simulink model "pacemaker_with_serial_communication"  (R2020b)
settings: Solver=FixedStepAuto  StartTime=0.0  StopTime=10.0  FixedStep=1e-3  RelTol=1e-3  EnableMultiTasking=on
undefined symbols (not defined in the file): A0, A1, D0, D1, D10, D11, D12, D13, D2, D3, D4, D5, D6, D7, D8, D9, PTA0, PTA1, PTA2, PTB2, PTB23, PTB3, PTB9, PTC16, PTC17, PTC2, PTC3, PTC4, PTD0, PTD1, PTD2, PTD3
libraries: frdmk64flib x21, etargetslib x17
settings Model: ExtModeTrigDuration=5  Creator=Anna  LastModifiedBy=Nafi
settings OptimizationCC: EnhancedBackFolding=on  PassReuseOutputArgsAs=Individual arguments  ZeroExternalMemoryAtStartup=off  ZeroInternalMemoryAtStartup=off  MaxStackSize=64  OptimizeBlockOrder=speed  DifferentSizesBufferReuse=on  OptimizationCustomize=off  EfficientTunableParamExpr=on
settings DebuggingCC: ParameterTunabilityLossMsg=error
settings HardwareCC: ProdBitPerPointer=32  ProdBitPerSizeT=32  ProdBitPerPtrDiffT=32  ProdLargestAtomicInteger=Long  ProdLargestAtomicFloat=Double  ProdWordSize=32  ProdHWDeviceType=ARM Compatible->ARM Cortex
settings SFSimCC: MATLABDynamicMemAlloc=off
settings RTWCC: Description=Embedded Coder  SystemTargetFile=ert.tlc  HardwareBoard=NXP FRDM-K64F  TLCOptions="-aInlineSetEventsForThisBaseRateFcn=TLC_FALSE -aSuppressMultiTaskScheduler=TLC_FALSE  -aRateBasedStepFcn=0"  TemplateMakefile=ert_default_tmf  Toolchain=GNU Tools for ARM Embedded Processors
settings CodeAppCC: ForceParamTrailComments=on  IgnoreCustomStorageClasses=off  OperatorAnnotations=on  SimulinkDataObjDesc=on  SFDataObjDesc=on  InsertBlockDesc=on
settings ERTTargetCC: ExtModeTransport=4  ExtModeMexFile=sendToCommService

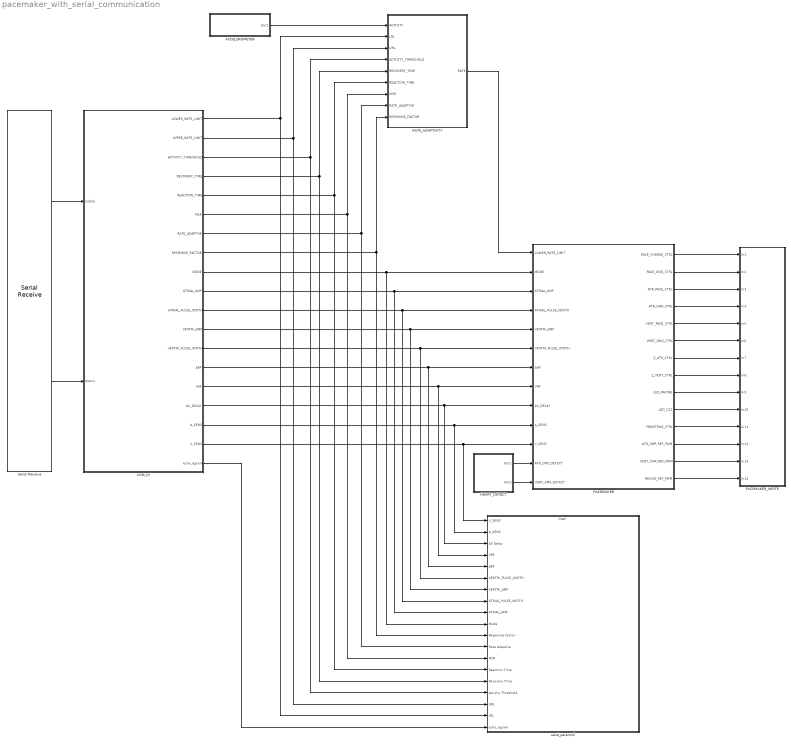
== system pacemaker_with_serial_communication ==
  ACCELEROMETER : Subsystem
  COM_IN : Stateflow chart  TreatAsAtomicUnit=on
      settings: PortSchema="{\"entries\":[{\"content\":{\"sides\":[{\"content\":{\"connectorIds\":[\"In1\",\"In2\"]},\"type\":\"ConnectorPlacement.EquallySpacedRectSide\",\"uuid\":\"cd1265d4-eeab-406f-839b-31637b64935e\"},{\"content\":{\"connectorIds\":[\"Out1\",\"Out2\",\"Out3\",\"Out4\",\"Out5\",\"Out6\",\"Out7\",\"Out8\",\"Out11\",\"Out15\",\"Out18\",\"Out16\",\"Out17\",\"Out10\",\"Out9\",\"Out13\",\"Out12\",\"Out14\",\"Out19\"],\"side\":\"RIGHT\"},\"type\":\"ConnectorPlacement.EquallySpacedRectSide\",\"uuid\":\"4c8a5d3b-ca50-43d3-bdc9-bcde3c420f64\"},{\"content\":{\"connectorIds\":[],\"side\":\"TOP\"},\"type\":\"ConnectorPlacement.EquallySpacedRectSide\",\"uuid\":\"7503811e-7a3c-4f49-863d-267d8f14587a\"},{\"content\":{\"connectorIds\":[],\"side\":\"HIDDEN\"},\"type\":\"ConnectorPlacement.EquallySpacedRectSide\",\"uuid\":\"b2e57f36-2a2e-483e-a972-25b3276b1e9d\"}]},\"type\":\"ConnectorPlacement.EquallySpacedConnector\",\"uuid\":\"ec734eff-85b8-4214-815d-279c5f21987a\"}],\"packageUris\":[\"http://schema.mathworks.com/mf0/Connector/R2020b\"],\"version\":\"1.0\"}"
  HEART_DETECT : Subsystem
  PACEMAKER : Stateflow chart  TreatAsAtomicUnit=on
      settings: PortSchema="{\"entries\":[{\"content\":{\"sides\":[{\"content\":{\"connectorIds\":[\"In2\",\"In1\",\"In3\",\"In4\",\"In5\",\"In6\",\"In7\",\"In8\",\"In9\",\"In10\",\"In11\",\"In12\",\"In13\"]},\"type\":\"ConnectorPlacement.EquallySpacedRectSide\",\"uuid\":\"703ea547-b5e3-494b-9c56-53f76044caab\"},{\"content\":{\"connectorIds\":[\"Out1\",\"Out2\",\"Out3\",\"Out4\",\"Out5\",\"Out6\",\"Out7\",\"Out8\",\"Out9\",\"Out10\",\"Out11\",\"Out12\",\"Out13\",\"Out14\"],\"side\":\"RIGHT\"},\"type\":\"ConnectorPlacement.EquallySpacedRectSide\",\"uuid\":\"cc2727a3-7e1d-4420-9643-b4757eb365ba\"},{\"content\":{\"connectorIds\":[],\"side\":\"TOP\"},\"type\":\"ConnectorPlacement.EquallySpacedRectSide\",\"uuid\":\"492b7801-5c9e-4474-b04e-880113f9bc08\"},{\"content\":{\"connectorIds\":[],\"side\":\"HIDDEN\"},\"type\":\"ConnectorPlacement.EquallySpacedRectSide\",\"uuid\":\"c524ea30-cb2c-406f-8230-58907bd7faf1\"}]},\"type\":\"ConnectorPlacement.EquallySpacedConnector\",\"uuid\":\"90428471-58b8-4273-9dd0-f9ed52ecca6a\"}],\"packageUris\":[\"http://schema.mathworks.com/mf0/Connector/R2020b\"],\"version\":\"1.0\"}"
  PACEMAKER_WRITE : Subsystem
  RATE_ADAPTIVITY : Stateflow chart  TreatAsAtomicUnit=on
      settings: PortSchema="{\"entries\":[{\"content\":{\"sides\":[{\"content\":{\"connectorIds\":[\"In1\",\"In2\",\"In3\",\"In4\",\"In6\",\"In5\",\"In7\",\"In8\",\"In9\"]},\"type\":\"ConnectorPlacement.EquallySpacedRectSide\",\"uuid\":\"d09d22a4-3bf2-447a-b888-9ed1bc13e508\"},{\"content\":{\"connectorIds\":[\"Out1\"],\"side\":\"RIGHT\"},\"type\":\"ConnectorPlacement.EquallySpacedRectSide\",\"uuid\":\"e5a6e6ed-c47a-4985-9dbc-dfef5f432796\"},{\"content\":{\"connectorIds\":[],\"side\":\"TOP\"},\"type\":\"ConnectorPlacement.EquallySpacedRectSide\",\"uuid\":\"14194fe3-110c-41d4-af12-2dfde4f1ce34\"},{\"content\":{\"connectorIds\":[],\"side\":\"HIDDEN\"},\"type\":\"ConnectorPlacement.EquallySpacedRectSide\",\"uuid\":\"89c167d3-ea6f-444e-9874-109804893e2e\"}]},\"type\":\"ConnectorPlacement.EquallySpacedConnector\",\"uuid\":\"492e352f-68f6-4e08-ae59-46af104c6e80\"}],\"packageUris\":[\"http://schema.mathworks.com/mf0/Connector/R2020b\"],\"version\":\"1.0\"}"
  Serial Receive : frdmk64flib/Serial Receive  SCIModule=0  Baudrate=uint32(9600)  Parity=None  StopBits=1  HardwareFlowControl=None  ByteOrder=LittleEndian  DataType=uint8  DataLength=52  BlockingMode=off  OutputStatus=on  SampleTime=0.015
  send_params() : Subsystem
  wires:
  COM_IN/17(VENTRI_PULSE_WIDTH) -> send_params()/6(VENTRI_PULSE_WIDTH), PACEMAKER/6(VENTRI_PULSE_WIDTH)
  COM_IN/10(ARP) -> send_params()/5(ARP), PACEMAKER/7(ARP)
  COM_IN/18(ATRIAL_PULSE_WIDTH) -> send_params()/8(ATRIAL_PULSE_WIDTH), PACEMAKER/4(ATRIAL_PULSE_WIDTH)
  COM_IN/12(A_SENS) -> send_params()/2(A_SENS), PACEMAKER/10(A_SENS)
  COM_IN/9(VRP) -> send_params()/4(VRP), PACEMAKER/8(VRP)
  COM_IN/1(LOWER_RATE_LIMIT) -> send_params()/18(LRL), RATE_ADAPTIVITY/2(LRL)
  COM_IN/13(AV_DELAY) -> send_params()/3(AV Delay), PACEMAKER/9(AV_DELAY)
  COM_IN/14(V_SENS) -> send_params()/1(V_SENS), PACEMAKER/11(V_SENS)
  COM_IN/11(MODE) -> send_params()/10(Mode), PACEMAKER/1(MODE)
  COM_IN/3(ACTIVITY_THRESHOLD) -> send_params()/16(Activity Threshold), RATE_ADAPTIVITY/4(ACTIVITY_THRESHOLD)
  COM_IN/6(MSR) -> send_params()/13(MSR), RATE_ADAPTIVITY/7(MSR)
  COM_IN/2(UPPER_RATE_LIMIT) -> send_params()/17(URL), RATE_ADAPTIVITY/3(URL)
  PACEMAKER/3(ATR_PACE_CTRL) -> PACEMAKER_WRITE/3(In3)
  COM_IN/7(RATE_ADAPTIVE) -> send_params()/12(Rate Adaptive), RATE_ADAPTIVITY/8(RATE_ADAPTIVE)
  RATE_ADAPTIVITY/1(RATE) -> PACEMAKER/2(LOWER_RATE_LIMIT)
  Serial Receive/2 -> COM_IN/2(status)
  PACEMAKER/9(LED_PACING) -> PACEMAKER_WRITE/9(In9)
  Serial Receive/1 -> COM_IN/1(rxdata)
  COM_IN/15(ATRIAL_AMP) -> send_params()/9(ATRIAL_AMP), PACEMAKER/3(ATRIAL_AMP)
  PACEMAKER/11(FRONTEND_CTRL) -> PACEMAKER_WRITE/11(In11)
  PACEMAKER/12(ATR_CMP_REF_PWM) -> PACEMAKER_WRITE/12(In12)
  PACEMAKER/1(PACE_CHARGE_CTRL) -> PACEMAKER_WRITE/1(In1)
  PACEMAKER/7(Z_ATR_CTRL) -> PACEMAKER_WRITE/7(In7)
  PACEMAKER/5(VENT_PACE_CTRL) -> PACEMAKER_WRITE/5(In5)
  PACEMAKER/10(LED_C22) -> PACEMAKER_WRITE/10(In10)
  PACEMAKER/2(PACE_GND_CTRL) -> PACEMAKER_WRITE/2(In2)
  PACEMAKER/14(PACING_REF_PWM) -> PACEMAKER_WRITE/14(In14)
  HEART_DETECT/2(Out2) -> PACEMAKER/13(VENT_CMP_DETECT)
  PACEMAKER/6(VENT_GND_CTRL) -> PACEMAKER_WRITE/6(In6)
  COM_IN/8(RESPONSE_FACTOR) -> send_params()/11(Response Factor), RATE_ADAPTIVITY/9(RESPONSE_FACTOR)
  PACEMAKER/4(ATR_GND_CTRL) -> PACEMAKER_WRITE/4(In4)
  COM_IN/5(REACTION_TIME) -> send_params()/14(Reaction Time), RATE_ADAPTIVITY/5(REACTION_TIME)
  COM_IN/16(VENTRI_AMP) -> send_params()/7(VENTRI_AMP), PACEMAKER/5(VENTRI_AMP)
  PACEMAKER/8(Z_VENT_CTRL) -> PACEMAKER_WRITE/8(In8)
  PACEMAKER/13(VENT_CMP_REF_PWM) -> PACEMAKER_WRITE/13(In13)
  COM_IN/4(RECOVERY_TIME) -> send_params()/15(Recovery Time), RATE_ADAPTIVITY/6(RECOVERY_TIME)
  HEART_DETECT/1(Out1) -> PACEMAKER/12(ATR_CMP_DETECT)
  COM_IN/19(echo_egram) -> send_params()/19(echo_egram)
  ACCELEROMETER/1(Out1) -> RATE_ADAPTIVITY/1(ACTIVITY)

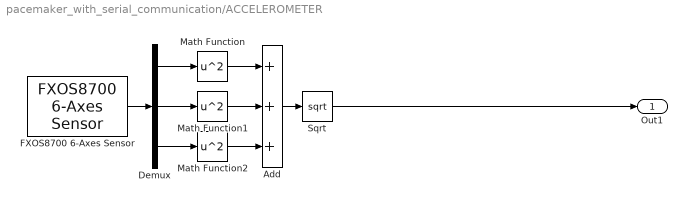
== system pacemaker_with_serial_communication/ACCELEROMETER ==
  Add : Sum  Inputs=+++
  Demux : Demux  Outputs=3
  FXOS8700 6-Axes Sensor : frdmk64flib/FXOS8700 6-Axes Sensor  Activesensor=Accelerometer only  ODR=800Hz  HybridODR=400Hz  Accelfullrange=-4g to +4g  SampleTime=-1
  Math Function : Math  Operator=square  SaturateOnIntegerOverflow=on
  Math Function1 : Math  Operator=square  SaturateOnIntegerOverflow=on
  Math Function2 : Math  Operator=square  SaturateOnIntegerOverflow=on
  Sqrt : Sqrt  SaturateOnIntegerOverflow=on
  Out1 : Outport
  wires:
  Add/1 -> Sqrt/1
  Demux/2 -> Math Function1/1
  Demux/3 -> Math Function2/1
  FXOS8700 6-Axes Sensor/1 -> Demux/1
  Demux/1 -> Math Function/1
  Math Function2/1 -> Add/3
  Sqrt/1 -> Out1/1
  Math Function/1 -> Add/1
  Math Function1/1 -> Add/2

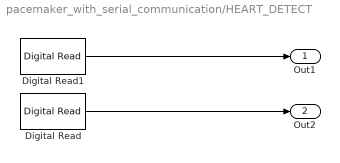
== system pacemaker_with_serial_communication/HEART_DETECT ==
  Digital Read : frdmk64flib/Digital Read  Whichpin=PTC17 (D1)  SampleTime=-1
  Digital Read1 : frdmk64flib/Digital Read  Whichpin=PTC16 (D0)  SampleTime=-1
  Out1 : Outport
  Out2 : Outport  Port=2
  wires:
  Digital Read/1 -> Out2/1
  Digital Read1/1 -> Out1/1

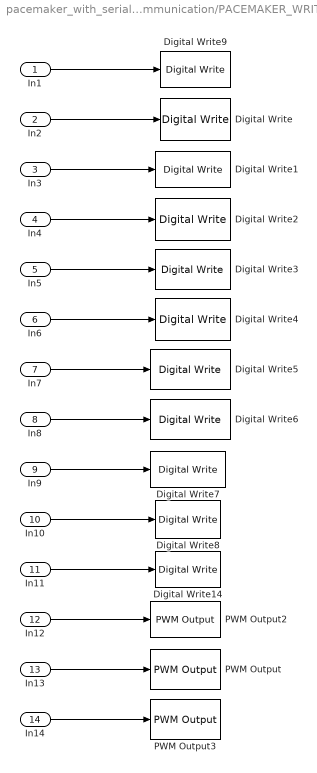
== system pacemaker_with_serial_communication/PACEMAKER_WRITE ==
  In1 : Inport
  In2 : Inport  Port=2
  In3 : Inport  Port=3
  In4 : Inport  Port=4
  In5 : Inport  Port=5
  In6 : Inport  Port=6
  In7 : Inport  Port=7
  In8 : Inport  Port=8
  In9 : Inport  Port=9
  In10 : Inport  Port=10
  In11 : Inport  Port=11
  In12 : Inport  Port=12
  In13 : Inport  Port=13
  In14 : Inport  Port=14
  Digital Write : frdmk64flib/Digital Write  Whichpin=PTD0 (D10)
  Digital Write1 : frdmk64flib/Digital Write  Whichpin=PTA0 (D8)
  Digital Write14 : frdmk64flib/Digital Write  Whichpin=PTD1 (D13)
  Digital Write2 : frdmk64flib/Digital Write  Whichpin=PTD2 (D11)
  Digital Write3 : frdmk64flib/Digital Write  Whichpin=PTC4 (D9)
  Digital Write4 : frdmk64flib/Digital Write  Whichpin=PTD3 (D12)
  Digital Write5 : frdmk64flib/Digital Write  Whichpin=PTB23 (D4)
  Digital Write6 : frdmk64flib/Digital Write  Whichpin=PTC3 (D7)
  Digital Write7 : frdmk64flib/Digital Write  Whichpin=RED_LED
  Digital Write8 : frdmk64flib/Digital Write  Whichpin=BLUE_LED
  Digital Write9 : frdmk64flib/Digital Write  Whichpin=PTB9 (D2)
  PWM Output : frdmk64flib/PWM Output  Whichpin=PTA1 (D3)  InitialFrequency=2000  InitialDutyCycle=100
  PWM Output2 : frdmk64flib/PWM Output  Whichpin=PTC2 (D6)  InitialFrequency=2000  InitialDutyCycle=100
  PWM Output3 : frdmk64flib/PWM Output  Whichpin=PTA2 (D5)  InitialFrequency=2000  InitialDutyCycle=100
  wires:
  In10/1 -> Digital Write8/1
  In2/1 -> Digital Write/1
  In12/1 -> PWM Output2/1
  In7/1 -> Digital Write5/1
  In4/1 -> Digital Write2/1
  In8/1 -> Digital Write6/1
  In11/1 -> Digital Write14/1
  In1/1 -> Digital Write9/1
  In6/1 -> Digital Write4/1
  In9/1 -> Digital Write7/1
  In14/1 -> PWM Output3/1
  In3/1 -> Digital Write1/1
  In13/1 -> PWM Output/1
  In5/1 -> Digital Write3/1

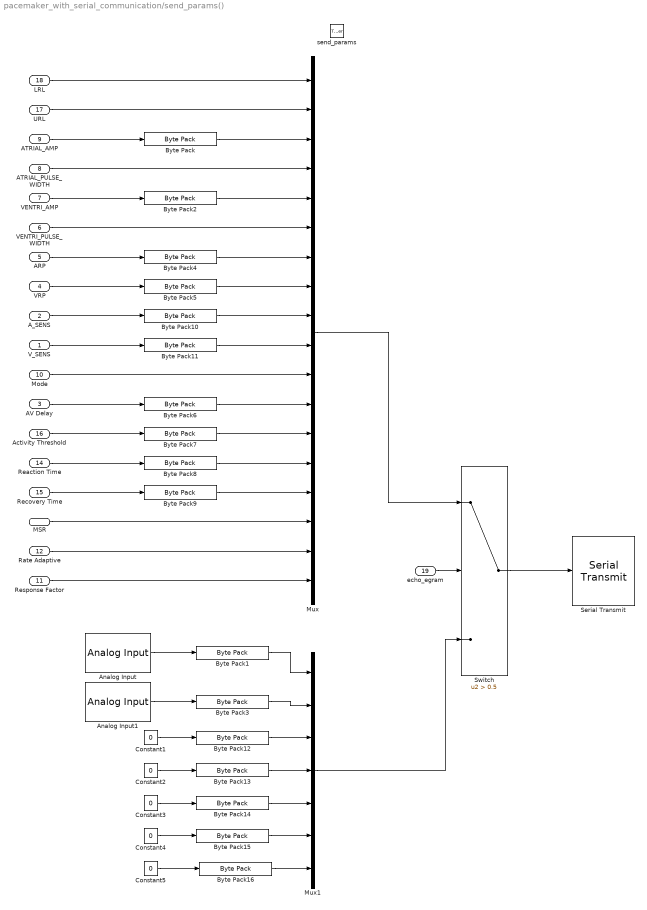
== system pacemaker_with_serial_communication/send_params() ==
  V_SENS : Inport
  A_SENS : Inport  Port=2
  AV Delay : Inport  Port=3
  VRP : Inport  Port=4
  ARP : Inport  Port=5
  VENTRI_PULSE_WIDTH : Inport  Port=6
  VENTRI_AMP : Inport  Port=7
  ATRIAL_PULSE_WIDTH : Inport  Port=8
  ATRIAL_AMP : Inport  Port=9
  Mode : Inport  Port=10
  Response Factor : Inport  Port=11
  Rate Adaptive : Inport  Port=12
  MSR : Inport  Port=13
  Reaction Time : Inport  Port=14
  Recovery Time : Inport  Port=15
  Activity Threshold : Inport  Port=16
  URL : Inport  Port=17
  LRL : Inport  Port=18
  echo_egram : Inport  Port=19
  send_params : TriggerPort  TriggerType=function-call  IsSimulinkFunction=on  FunctionName=send_params  VariantControl=Variant
  Analog Input : frdmk64flib/Analog Input  Whichpin=PTB2 (A0)  SampleTime=-1
  Analog Input1 : frdmk64flib/Analog Input  Whichpin=PTB3 (A1)  SampleTime=-1
  Byte Pack{,2,7,10..11} (5 alike) : etargetslib/Byte Pack  datatypes={'single'}  byteAlign=1
  Byte Pack{1,3,8..9,12..15} (8 alike) : etargetslib/Byte Pack  datatypes={'double'}  byteAlign=1
  Byte Pack{4..6,16} (4 alike) : etargetslib/Byte Pack  datatypes={'uint16'}  byteAlign=1
  Constant{1..4} (4 alike) : Constant  Value=0  OutDataTypeStr=double
  Constant5 : Constant  Value=0  OutDataTypeStr=uint16
  Mux : Mux  Inputs=18
  Mux1 : Mux  Inputs=7
  Serial Transmit : frdmk64flib/Serial Transmit  SCIModule=0  Baudrate=uint32(9600)  Parity=None  StopBits=1  HardwareFlowControl=None  ByteOrder=LittleEndian  BlockingMode=on  OutputStatus=off
  Switch : Switch  Criteria=u2 > Threshold  Threshold=0.5
  wires:
  LRL/1 -> Mux/1
  URL/1 -> Mux/2
  ATRIAL_AMP/1 -> Byte Pack/1
  VENTRI_AMP/1 -> Byte Pack2/1
  ARP/1 -> Byte Pack4/1
  VRP/1 -> Byte Pack5/1
  A_SENS/1 -> Byte Pack10/1
  AV Delay/1 -> Byte Pack6/1
  Activity Threshold/1 -> Byte Pack7/1
  Reaction Time/1 -> Byte Pack8/1
  Recovery Time/1 -> Byte Pack9/1
  Byte Pack/1 -> Mux/3
  ATRIAL_PULSE_WIDTH/1 -> Mux/4
  Byte Pack2/1 -> Mux/5
  VENTRI_PULSE_WIDTH/1 -> Mux/6
  Byte Pack4/1 -> Mux/7
  Byte Pack5/1 -> Mux/8
  V_SENS/1 -> Byte Pack11/1
  Byte Pack10/1 -> Mux/9
  Analog Input/1 -> Byte Pack1/1
  Analog Input1/1 -> Byte Pack3/1
  Constant1/1 -> Byte Pack12/1
  Constant2/1 -> Byte Pack13/1
  Constant3/1 -> Byte Pack14/1
  Constant4/1 -> Byte Pack15/1
  Constant5/1 -> Byte Pack16/1
  Byte Pack15/1 -> Mux1/6
  Byte Pack14/1 -> Mux1/5
  Byte Pack13/1 -> Mux1/4
  Byte Pack12/1 -> Mux1/3
  Byte Pack1/1 -> Mux1/1
  Byte Pack3/1 -> Mux1/2
  echo_egram/1 -> Switch/2
  Mux1/1 -> Switch/3
  Mux/1 -> Switch/1
  Switch/1 -> Serial Transmit/1
  Byte Pack16/1 -> Mux1/7
  Byte Pack11/1 -> Mux/10
  Mode/1 -> Mux/11
  Byte Pack9/1 -> Mux/15
  Byte Pack6/1 -> Mux/12
  Byte Pack7/1 -> Mux/13
  Byte Pack8/1 -> Mux/14
  MSR/1 -> Mux/16
  Rate Adaptive/1 -> Mux/17
  Response Factor/1 -> Mux/18

== stateflow chart pacemaker_with_serial_communication/COM_IN ==
  settings: executeAtInitialization=1
  state SET_PARAMS
    entry:
    LOWER_RATE_LIMIT = rxdata(3)
    UPPER_RATE_LIMIT = rxdata(4)
    ATRIAL_AMP = typecast(rxdata(5:8), 'single')
    ATRIAL_PULSE_WIDTH = rxdata(9)
    VENTRI_AMP = typecast(rxdata(10:13), 'single')
    VENTRI_PULSE_WIDTH = rxdata(14)
    ARP = typecast(rxdata(15:16), 'uint16')
    VRP = typecast(rxdata(17:18), 'uint16')
    A_SENS = typecast(rxdata(19:22), 'single')
    V_SENS = typecast(rxdata(23:26), 'single')
    MODE = rxdata(27)
    AV_DELAY = typecast(rxdata(28:29),'uint16')
    ACTIVITY_THRESHOLD = typecast(rxdata(30:33), 'single')
    REACTION_TIME = typecast(rxdata(34:41), 'double')
    RECOVERY_TIME = typecast(rxdata(42:49), 'double')
    MSR = rxdata(50)
    RATE_ADAPTIVE = rxdata(51)
    RESPONSE_FACTOR= rxdata(52)
  state INIT
    entry:
    LOWER_RATE_LIMIT = 30
    UPPER_RATE_LIMIT = 120
    ATRIAL_AMP = 5
    ATRIAL_PULSE_WIDTH = 10
    VENTRI_AMP = 5
    VENTRI_PULSE_WIDTH = 10
    ARP = 100
    VRP = 100
    A_SENS= 3
    V_SENS = 3
    MODE = 4
    AV_DELAY = 50
    ACTIVITY_THRESHOLD = 1.1
    REACTION_TIME = 2000
    RECOVERY_TIME = 2000
    MSR = 120
    RATE_ADAPTIVE= 1
    RESPONSE_FACTOR = 16
  state SEND_EGRAM
    entry:
    echo_egram = 0
    send_params()
  state STANDBY
  state SEND_PARAMS
    entry:
    echo_egram = 1
    send_params();
  SET_PARAMS -> STANDBY
  (junction 10) -> SET_PARAMS [order 2] : [rxdata(2) == hex2dec('55')]
  (default) -> INIT
  INIT -> STANDBY
  STANDBY -> (junction 10) : [status == 0 && rxdata(1) == hex2dec('16')]
  (junction 10) -> SEND_EGRAM [order 1] : [rxdata(2) == hex2dec('47')]
  (junction 10) -> SEND_PARAMS [order 3] : [rxdata(2) == hex2dec('22')]
  SEND_EGRAM -> STANDBY
  SEND_PARAMS -> STANDBY
  data: LOWER_RATE_LIMIT output uint8; rxdata input uint8; status input uint8; UPPER_RATE_LIMIT output uint8; ACTIVITY_THRESHOLD output single; RECOVERY_TIME output double; REACTION_TIME output double; MSR output uint8; RATE_ADAPTIVE output uint8; RESPONSE_FACTOR output uint8; VRP output uint16; ARP output uint16; MODE output uint8; A_SENS output single; AV_DELAY output uint16; V_SENS output single; ATRIAL_AMP output single; VENTRI_AMP output single; VENTRI_PULSE_WIDTH output uint8; ATRIAL_PULSE_WIDTH output uint8; echo_egram output

== stateflow chart pacemaker_with_serial_communication/RATE_ADAPTIVITY ==
  state MIN_RATE
    AVG_ACTIVITY = (AVG_ACTIVITY + ACTIVITY)/2
    if RATE > LRL
    RATE = RATE - (MSR-LRL)/RECOVERY_TIME
    DELAY = RECOVERY_TIME
    else
    RATE = LRL
    DELAY = 0
    end
  state INITIAL
    RATE = LRL
    AVG_ACTIVITY = ACTIVITY
  state RATE_ADAPTIVE_DEFAULT
  state RATE_ADAPTIVE
    ADJUSTED_RATE = (0.57*RESPONSE_FACTOR^2-1.34*RESPONSE_FACTOR+22.71)*(AVG_ACTIVITY- double(ACTIVITY_THRESHOLD))+LRL
    if ADJUSTED_RATE > MSR
    ADJUSTED_RATE = MSR
    elseif ADJUSTED_RATE < LRL
    ADJUSTED_RATE = LRL
    end
  state OFFSET
    AVG_ACTIVITY = (AVG_ACTIVITY + ACTIVITY)/2
    if RATE > ADJUSTED_RATE
    RATE = RATE - (MSR-LRL)/RECOVERY_TIME
    DELAY = RECOVERY_TIME
    elseif RATE < ADJUSTED_RATE
    RATE = RATE + (MSR-LRL)/REACTION_TIME
    DELAY = REACTION_TIME
    end
  MIN_RATE -> RATE_ADAPTIVE [order 1] : [n>= DELAY && AVG_ACTIVITY>=ACTIVITY_THRESHOLD]
  MIN_RATE -> MIN_RATE [order 2] : after(1,msec){n=n+1}
  MIN_RATE -> INITIAL [order 3] : [RATE_ADAPTIVE == 0 && n>=DELAY]
  RATE_ADAPTIVE_DEFAULT -> MIN_RATE [order 2] : [AVG_ACTIVITY < double(ACTIVITY_THRESHOLD)]{n=0}
  (default) -> INITIAL
  INITIAL -> RATE_ADAPTIVE_DEFAULT : [RATE_ADAPTIVE == 1]{ADJUSTED_RATE = RATE}
  RATE_ADAPTIVE_DEFAULT -> RATE_ADAPTIVE [order 1] : [AVG_ACTIVITY>= ACTIVITY_THRESHOLD]
  OFFSET -> RATE_ADAPTIVE_DEFAULT [order 1] : [n>=DELAY]
  RATE_ADAPTIVE -> OFFSET : {n=0, AVG_ACTIVITY = ACTIVITY}
  OFFSET -> OFFSET [order 2] : after(1, msec){n=n+1}
  data: ACTIVITY input; LRL input uint8; RATE output; URL input uint8; ACTIVITY_THRESHOLD input single; REACTION_TIME input double; RECOVERY_TIME input double; MSR input uint8; BPM_PREV local; CURRENT_BPM local; PREV_ACCEL local; n local; AVG_ACCEL local; RATE_ADAPTIVE input uint8; RESPONSE_FACTOR input uint8; ADJUSTED_RATE local; AVG_ACTIVITY local; DELAY local

== stateflow chart pacemaker_with_serial_communication/PACEMAKER ==
  state MODE_VVI [commented out]
    entry:
    FRONTEND_CTRL = true
    state VVI_CHARGING_SENSING [commented out]
      entry:
      %Sensing Circuitry
      VENT_CMP_REF_PWM = DUTY_CYCLE
      ATR_CMP_REF_PWM = 0
      %Discharging C21
      PACE_GND_CTRL = true
      VENT_PACE_CTRL = false
      Z_ATR_CTRL = false
      Z_VENT_CTRL = false
      ATR_PACE_CTRL = false
      ATR_GND_CTRL = false
      VENT_GND_CTRL = true
      %Charging C22
      ATR_PACE_CTRL = false
      VENT_PACE_CTRL = false
      PACING_REF_PWM = 100*VENTRI_AMP/5
      PACE_CHARGE_CTRL = true
      LED_C22 = true
      exit:
      LED_C22 = false
    state PACE_READY [commented out]
      entry:
      %Discharging C21
      PACE_GND_CTRL = true
      VENT_PACE_CTRL = false
      Z_ATR_CTRL = false
      Z_VENT_CTRL = false
      ATR_PACE_CTRL = false
      ATR_GND_CTRL = false
      VENT_GND_CTRL = true
      %Charging C22
      ATR_PACE_CTRL = false
      VENT_PACE_CTRL = false
      PACING_REF_PWM = 100*VENTRI_AMP/5
      PACE_CHARGE_CTRL = true
      LED_C22 = true
      exit:
      LED_C22 = false
    state PACING_VENTRICLE_VVI [commented out]
      entry:
      PACE_CHARGE_CTRL = false
      PACE_GND_CTRL = true
      ATR_PACE_CTRL = false
      ATR_GND_CTRL = false
      Z_ATR_CTRL = false
      Z_VENT_CTRL = false
      VENT_GND_CTRL = false
      VENT_PACE_CTRL = true
      LED_PACING = true
      exit:
      LED_PACING = false
    VVI_CHARGING_SENSING -> PACING_VENTRICLE_VVI [commented out] : after(((60000/LOWER_RATE_LIMIT)-VENTRI_PULSE_WIDTH-VRP),msec) [VENT_CMP_DETECT== false]
    (default) -> VVI_CHARGING_SENSING [commented out]
    MODE_VVI.PACE_READY -> VVI_CHARGING_SENSING [commented out] : after(VRP, msec)
    PACING_VENTRICLE_VVI -> MODE_VVI.PACE_READY [commented out] : after(VENTRI_PULSE_WIDTH, msec)
    VVI_CHARGING_SENSING -> MODE_VVI.PACE_READY [commented out] : [VENT_CMP_DETECT == true]
  state MODE_VOO [commented out]
    entry:
    FRONTEND_CTRL = false
    state VOO_CHARGING [commented out]
      entry:
      %Discharging C21
      PACE_GND_CTRL = true
      VENT_PACE_CTRL = false
      Z_ATR_CTRL = false
      Z_VENT_CTRL = false
      ATR_GND_CTRL = false
      ATR_PACE_CTRL = false
      VENT_GND_CTRL = true
      %Charging C22
      ATR_PACE_CTRL = false
      VENT_PACE_CTRL = false
      PACING_REF_PWM = 100*VENTRI_AMP/5
      PACE_CHARGE_CTRL = true
      LED_C22 = true
      exit:
      LED_C22 = false
    state PACING_VENTRICLE_VOO [commented out]
      entry:
      PACE_CHARGE_CTRL = false
      PACE_GND_CTRL = true
      ATR_PACE_CTRL = false
      ATR_GND_CTRL = false
      Z_ATR_CTRL = false
      Z_VENT_CTRL = false
      VENT_GND_CTRL = false
      VENT_PACE_CTRL = true
      LED_PACING = true
      exit:
      LED_PACING = false
    PACING_VENTRICLE_VOO -> VOO_CHARGING [commented out] : after(VENTRI_PULSE_WIDTH, msec)
    (default) -> VOO_CHARGING [commented out]
    VOO_CHARGING -> PACING_VENTRICLE_VOO [commented out] : after(((60000/LOWER_RATE_LIMIT)-VENTRI_PULSE_WIDTH), msec)
  state ATRIUM_CHARGING
    entry:
    %Sensing Circuitry
    FRONTEND_CTRL = true
    ATR_CMP_REF_PWM = 100*A_SENS/5
    %Discharging C21
    PACE_GND_CTRL = true
    VENT_PACE_CTRL = false
    Z_ATR_CTRL = false
    Z_VENT_CTRL = false
    ATR_PACE_CTRL = false
    ATR_GND_CTRL = true
    VENT_GND_CTRL = false
    %Charging C22
    ATR_PACE_CTRL = false
    VENT_PACE_CTRL = false
    PACING_REF_PWM = 100*ATRIAL_AMP/5
    PACE_CHARGE_CTRL = true
    LED_C22 = true
    exit:
    LED_C22 = false
  state VENTRICLE_CHARGING
    entry:
    %Sensing Circuitry
    FRONTEND_CTRL = true
    VENT_CMP_REF_PWM = 100*V_SENS/5
    %Discharging C21
    PACE_GND_CTRL = true
    VENT_PACE_CTRL = false
    Z_ATR_CTRL = false
    Z_VENT_CTRL = false
    ATR_PACE_CTRL = false
    ATR_GND_CTRL = false
    VENT_GND_CTRL = true
    %Charging C22
    ATR_PACE_CTRL = false
    VENT_PACE_CTRL = false
    PACING_REF_PWM = 100*VENTRI_AMP/5
    PACE_CHARGE_CTRL = true
    LED_C22 = true
    exit:
    LED_C22 = false
  state PACING_VENTRICLE
    entry:
    PACE_CHARGE_CTRL = false
    PACE_GND_CTRL = true
    ATR_PACE_CTRL = false
    ATR_GND_CTRL = false
    Z_ATR_CTRL = false
    Z_VENT_CTRL = false
    VENT_GND_CTRL = false
    VENT_PACE_CTRL = true
    LED_PACING = true
    exit:
    LED_PACING = false
  state PACING_ATRIUM
    entry:
    PACE_CHARGE_CTRL = false
    PACE_GND_CTRL = true
    ATR_PACE_CTRL = true
    ATR_GND_CTRL = false
    Z_ATR_CTRL = false
    Z_VENT_CTRL = false
    VENT_GND_CTRL = false
    VENT_PACE_CTRL = false
    LED_PACING = true
    exit:
    LED_PACING = false
  state INITIAL
    %initial state
  state MODE_AAI [commented out]
    entry:
    FRONTEND_CTRL = true
    state AAI_CHARGING_SENSING [commented out]
      entry:
      %Sensing Circuitry
      VENT_CMP_REF_PWM = 0
      ATR_CMP_REF_PWM = DUTY_CYCLE
      %Discharging C21
      PACE_GND_CTRL = true
      VENT_PACE_CTRL = false
      Z_ATR_CTRL = false
      Z_VENT_CTRL = false
      ATR_PACE_CTRL = false
      ATR_GND_CTRL = true
      VENT_GND_CTRL = false
      %Charging C22
      ATR_PACE_CTRL = false
      VENT_PACE_CTRL = false
      PACING_REF_PWM = 100*ATRIAL_AMP/5
      PACE_CHARGE_CTRL = true
      LED_C22 = true
      exit:
      LED_C22 = false
    state PACE_READY [commented out]
      entry:
      %Discharging C21
      PACE_GND_CTRL = true
      VENT_PACE_CTRL = false
      Z_ATR_CTRL = false
      Z_VENT_CTRL = false
      ATR_PACE_CTRL = false
      ATR_GND_CTRL = true
      VENT_GND_CTRL = false
      %Charging C22
      ATR_PACE_CTRL = false
      VENT_PACE_CTRL = false
      PACING_REF_PWM = 100*ATRIAL_AMP/5
      PACE_CHARGE_CTRL = true
      LED_C22 = true
      exit:
      LED_C22 = false
    state PACING_ATRIUM_AAI [commented out]
      entry:
      PACE_CHARGE_CTRL = false
      PACE_GND_CTRL = true
      ATR_PACE_CTRL = true
      ATR_GND_CTRL = false
      Z_ATR_CTRL = false
      Z_VENT_CTRL = false
      VENT_GND_CTRL = false
      VENT_PACE_CTRL = false
      LED_PACING = true
      exit:
      LED_PACING = false
    AAI_CHARGING_SENSING -> PACING_ATRIUM_AAI [commented out] : after(((60000/LOWER_RATE_LIMIT)-ATRIAL_PULSE_WIDTH-ARP),msec) [ATR_CMP_DETECT== false]
    (default) -> AAI_CHARGING_SENSING [commented out]
    MODE_AAI.PACE_READY -> AAI_CHARGING_SENSING [commented out] : after(ARP, msec)
    PACING_ATRIUM_AAI -> MODE_AAI.PACE_READY [commented out] : after(ATRIAL_PULSE_WIDTH, msec)
    AAI_CHARGING_SENSING -> MODE_AAI.PACE_READY [commented out] : [ATR_CMP_DETECT == true]
  state MODE_AOO [commented out]
    entry:
    FRONTEND_CTRL = false
    state AOO_CHARGING [commented out]
      entry:
      %Discharging C21
      PACE_GND_CTRL = true
      VENT_PACE_CTRL = false
      Z_ATR_CTRL = false
      Z_VENT_CTRL = false
      ATR_PACE_CTRL = false
      ATR_GND_CTRL = true
      VENT_GND_CTRL = false
      %Charging C22
      ATR_PACE_CTRL = false
      VENT_PACE_CTRL = false
      PACING_REF_PWM = 100*ATRIAL_AMP/5
      PACE_CHARGE_CTRL = true
      LED_C22 = true
      exit:
      LED_C22 = false
    state PACING_ATRIUM_AOO [commented out]
      entry:
      PACE_CHARGE_CTRL = false
      PACE_GND_CTRL = true
      ATR_PACE_CTRL = true
      ATR_GND_CTRL = false
      Z_ATR_CTRL = false
      Z_VENT_CTRL = false
      VENT_GND_CTRL = false
      VENT_PACE_CTRL = false
      LED_PACING = true
      exit:
      LED_PACING = false
    AOO_CHARGING -> PACING_ATRIUM_AOO [commented out] : after(((60000/LOWER_RATE_LIMIT)-ATRIAL_PULSE_WIDTH), msec)
    (default) -> AOO_CHARGING [commented out]
    PACING_ATRIUM_AOO -> AOO_CHARGING [commented out] : after(ATRIAL_PULSE_WIDTH, msec)
  state CHARGING_DOO_2
    entry:
    %Discharging C21 Atrium
    PACE_GND_CTRL = true
    VENT_PACE_CTRL = false
    Z_ATR_CTRL = false
    Z_VENT_CTRL = false
    ATR_GND_CTRL = false
    ATR_PACE_CTRL = true
    VENT_GND_CTRL = false
    %Charging C22 Ventricle
    ATR_PACE_CTRL = false
    VENT_PACE_CTRL = false
    PACING_REF_PWM = 100*VENTRI_AMP/5
    PACE_CHARGE_CTRL = true
    LED_C22 = true
    exit:
    LED_C22 = false
  state CHARGING_DOO
    entry:
    %Discharging C21 Ventricle
    PACE_GND_CTRL = true
    VENT_PACE_CTRL = false
    Z_ATR_CTRL = false
    Z_VENT_CTRL = false
    ATR_GND_CTRL = false
    ATR_PACE_CTRL = false
    VENT_GND_CTRL = true
    %Charging C22 Atrium
    ATR_PACE_CTRL = false
    VENT_PACE_CTRL = false
    PACING_REF_PWM = 100*ATRIAL_AMP/5
    PACE_CHARGE_CTRL = true
    LED_C22 = true
    exit:
    LED_C22 = false
  state PACING_ATRIUM_DOO
    entry:
    PACE_CHARGE_CTRL = false
    PACE_GND_CTRL = true
    ATR_PACE_CTRL = true
    ATR_GND_CTRL = false
    Z_ATR_CTRL = false
    Z_VENT_CTRL = false
    VENT_GND_CTRL = false
    VENT_PACE_CTRL = false
    LED_PACING = true
    exit:
    LED_PACING = false
  state PACING_VENTRICLE_DOO
    entry:
    PACE_CHARGE_CTRL = false
    PACE_GND_CTRL = true
    ATR_PACE_CTRL = false
    ATR_GND_CTRL = false
    Z_ATR_CTRL = false
    Z_VENT_CTRL = false
    VENT_GND_CTRL = false
    VENT_PACE_CTRL = true
    LED_PACING = true
    exit:
    LED_PACING = false
  VENTRICLE_CHARGING -> ATRIUM_CHARGING [order 3] : [MODE == 0 || MODE == 2]
  ATRIUM_CHARGING -> VENTRICLE_CHARGING [order 3] : [MODE == 1 || MODE == 3]
  VENTRICLE_CHARGING -> PACING_VENTRICLE [order 1] : after(((60000/LOWER_RATE_LIMIT)-VENTRI_PULSE_WIDTH), msec)
  ATRIUM_CHARGING -> PACING_ATRIUM [order 1] : after(((60000/LOWER_RATE_LIMIT)-ATRIAL_PULSE_WIDTH), msec)
  INITIAL -> ATRIUM_CHARGING [order 1] : [MODE == 0 || MODE == 2]
  (junction 79) -> MODE_VOO [commented out] : [MODE == 1]
  INITIAL -> VENTRICLE_CHARGING [order 2] : [MODE == 1 || MODE == 3]
  (junction 79) -> MODE_VVI [commented out]
  (default) -> INITIAL
  (default) -> (junction 79) [commented out]
  INITIAL -> CHARGING_DOO [order 3] : [MODE == 4]
  PACING_ATRIUM -> ATRIUM_CHARGING : after(ATRIAL_PULSE_WIDTH, msec)
  PACING_VENTRICLE -> VENTRICLE_CHARGING : after(VENTRI_PULSE_WIDTH, msec)
  (junction 79) -> MODE_AAI [commented out] : [MODE == 2]
  (junction 79) -> MODE_AOO [commented out] : [MODE == 0]
  VENTRICLE_CHARGING -> VENTRICLE_CHARGING [order 2] : after(VRP,msec) [MODE ==3 && VENT_CMP_DETECT == true]
  CHARGING_DOO_2 -> VENTRICLE_CHARGING [order 2] : [MODE == 1 || MODE == 3]
  CHARGING_DOO -> ATRIUM_CHARGING [order 2] : [MODE == 0 || MODE == 2]
  ATRIUM_CHARGING -> ATRIUM_CHARGING [order 2] : after(ARP,msec) [MODE == 2 && ATR_CMP_DETECT == true]
  CHARGING_DOO -> PACING_ATRIUM_DOO [order 1] : after((uint16((60000/LOWER_RATE_LIMIT)-VENTRI_PULSE_WIDTH)-(AV_DELAY)), msec)
  PACING_ATRIUM_DOO -> CHARGING_DOO_2 : after(ATRIAL_PULSE_WIDTH, msec)
  CHARGING_DOO_2 -> PACING_VENTRICLE_DOO [order 1] : after((AV_DELAY-uint16(ATRIAL_PULSE_WIDTH)), msec)
  PACING_VENTRICLE_DOO -> CHARGING_DOO : after(VENTRI_PULSE_WIDTH, msec)
  data: MODE input uint8; PACE_CHARGE_CTRL output; PACE_GND_CTRL output; ATR_PACE_CTRL output; ATR_GND_CTRL output; VENT_PACE_CTRL output; VENT_GND_CTRL output; Z_ATR_CTRL output; Z_VENT_CTRL output; LED_PACING output; LED_C22 output; LOWER_RATE_LIMIT input uint8; ATRIAL_AMP input single; ATRIAL_PULSE_WIDTH input uint8; VENTRI_AMP input single; VENTRI_PULSE_WIDTH input uint8; ARP input uint16; VRP input uint16; FRONTEND_CTRL output; ATR_CMP_REF_PWM output; VENT_CMP_REF_PWM output; PACING_REF_PWM output; AV_DELAY input uint16; A_SENS input single; V_SENS input single; ATR_CMP_DETECT input; VENT_CMP_DETECT input
